simulink model "ExoskeletonControlModel"  (R2022b)
settings: Solver=ode3  StartTime=0.0  StopTime=inf  FixedStep=Ts  RelTol=1e-3
PreLoadFcn:
  | Ts_IO204 = 0.001;
  | 
  | if ~exist('Ts', 'var')
  | Ts = 0.001;
  | end
  | if ~exist('FPGA_Frequency', 'var')
  | FPGA_Frequency = 75000000;
  | end
  | 
  | ts_IO612 = 1e-3;
  | 
  | load('TargetReached.mat')
  | load('ActualPos_inc.mat')
model workspace (MAT data in the model file):
  DeltaData = timeseries
  DeltaData.DataInfo = tsdata.datametadata
  DeltaData.DataInfo.Interpolation = tsdata.interpolation
  DeltaData.DataInfo.Interpolation.Fhandle : function handle (value not decoded)
  DeltaData.DataInfo.Interpolation.Name = 'linear'
  DeltaData.TimeInfo = tsdata.timemetadata
  DeltaData.TimeInfo.Length = 30001
  DeltaData.TimeInfo.DuplicateTimes = 0
  DeltaData.TimeInfo.Increment_ = 0.001
  DeltaData.TimeInfo.Start_ = 0
  DeltaData.TimeInfo.Initialized = 1
  DeltaData.QualityInfo = tsdata.qualmetadata
  DeltaData.Data_ = [0 0 0 0 0 0 0 0 0 0 0 0 ... (180006 elements, 6x1x30001)]
  DeltaData.IsTimeFirst_ = 0
  EC45_deg2incs = 2276
  EC60_deg2inc = 5461
  EC90_deg2incs = 7111
  Enc2rad_18bit = 2.3968e-05
  Enc2rad_19bit = 1.1984e-05
  Enc2rad_20bit = 5.9921e-06
  GiulioModel = robotics.RigidBodyTree
  GiulioModel.TreeInternal = robotics.manip.internal.RigidBodyTree
  GiulioModel.TreeInternal.NumBodies = 7
  GiulioModel.TreeInternal.Base = robotics.manip.internal.RigidBody
  GiulioModel.TreeInternal.Base.Index = 0
  GiulioModel.TreeInternal.Base.NameInternal = 'base'
  GiulioModel.TreeInternal.Base.JointInternal = robotics.Joint
  GiulioModel.TreeInternal.Base.JointInternal.Type = 'fixed'
  GiulioModel.TreeInternal.Base.JointInternal.VelocityNumber = 0
  GiulioModel.TreeInternal.Base.JointInternal.PositionNumber = 0
  GiulioModel.TreeInternal.Base.JointInternal.MotionSubspace = [0; 0; 0; 0; 0; 0]
  GiulioModel.TreeInternal.Base.JointInternal.NameInternal = 'base_jnt'
  GiulioModel.TreeInternal.Base.ParentIndex = -1
  GiulioModel.TreeInternal.Base.ChildrenIndices = 1
  GiulioModel.TreeInternal.Base.MassInternal = 1
  GiulioModel.TreeInternal.Base.CenterOfMassInternal = [0 0 0]
  GiulioModel.TreeInternal.Base.InertiaInternal = [1  0  0; 0  1  0; 0  0  1]
  GiulioModel.TreeInternal.Base.SpatialInertia = [1  0  0  0  0  0; 0  1  0  0  0  0; 0  0  1  0  0  0; 0  0  0  1  0  0; 0  0  0  0  1  0; 0  0  0  0  0  1]
  GiulioModel.TreeInternal.Base.CollisionsInternal = robotics.manip.internal.CollisionSet
  GiulioModel.TreeInternal.Base.CollisionsInternal.MaxElements = 0
  GiulioModel.TreeInternal.FastVisualizationHelper = robotics.manip.internal.FastVisualizationHelper
  GiulioModel.TreeInternal.FastVisualizationHelper.IsUpdated = 0
  GiulioModel.TreeInternal.FastVisualizationHelper.MeshAndFrameOptions = [0 1 1]
  GiulioModel.TreeInternal.Gravity = [0 0 -9.81]
  GiulioModel.TreeInternal.Bodies{1} = robotics.manip.internal.RigidBody
  GiulioModel.TreeInternal.Bodies{1}.Index = 1
  GiulioModel.TreeInternal.Bodies{1}.NameInternal = 'body1'
  GiulioModel.TreeInternal.Bodies{1}.JointInternal = robotics.Joint
  GiulioModel.TreeInternal.Bodies{1}.JointInternal.Type = 'revolute'
  GiulioModel.TreeInternal.Bodies{1}.JointInternal.VelocityNumber = 1
  GiulioModel.TreeInternal.Bodies{1}.JointInternal.PositionNumber = 1
  GiulioModel.TreeInternal.Bodies{1}.JointInternal.MotionSubspace = [0; 0; 1; 0; 0; 0]
  GiulioModel.TreeInternal.Bodies{1}.JointInternal.InTree = 1
  GiulioModel.TreeInternal.Bodies{1}.JointInternal.JointToParentTransform = [1  0  0  0; 0  -1  -1.22464679915e-16  0; 0  1.22464679915e-16  -1  0; 0  0  0  1]
  GiulioModel.TreeInternal.Bodies{1}.JointInternal.NameInternal = 'jnt1'
  GiulioModel.TreeInternal.Bodies{1}.JointInternal.PositionLimitsInternal = [-0.733038285838 0.767246739177]
  GiulioModel.TreeInternal.Bodies{1}.JointInternal.JointAxisInternal = [0 0 1]
  GiulioModel.TreeInternal.Bodies{1}.ParentIndex = 0
  GiulioModel.TreeInternal.Bodies{1}.ChildrenIndices = [0 1]
  GiulioModel.TreeInternal.Bodies{1}.MassInternal = 2.789186
  GiulioModel.TreeInternal.Bodies{1}.CenterOfMassInternal = [5.3227185e-05 0.0036472886 -0.10689989]
  GiulioModel.TreeInternal.Bodies{1}.InertiaInternal = [0.010235641  5.0405441e-06  1.1186417e-05; 5.0405441e-06  0.011235393  0.0013102424; 1.1186417e-05  0.0013102424  0.0033699993]
  GiulioModel.TreeInternal.Bodies{1}.SpatialInertia = [0.010235641  5.0405441e-06  1.1186417e-05  0  0.29816367659  0.0101729663011; 5.0405441e-06  0.011235393  0.0013102424  -0.29816367659  0  -0.000148460519221; 1.1186417e-05  0.0013102424  0.0033699993  -0.0101729663011  0.000148460519221  0; 0  -0.29816367659  -0.0101729663011  2.789186  0  0; 0.29816367659  0  0.000148460519221  0  2.789186  0; 0.0101729663011  -0.000148460519221  0  0  0  2.789186]
  GiulioModel.TreeInternal.Bodies{1}.CollisionsInternal = robotics.manip.internal.CollisionSet
  GiulioModel.TreeInternal.Bodies{1}.CollisionsInternal.MaxElements = 0
  GiulioModel.TreeInternal.Bodies{2} = robotics.manip.internal.RigidBody
  GiulioModel.TreeInternal.Bodies{2}.Index = 2
  GiulioModel.TreeInternal.Bodies{2}.NameInternal = 'body2'
  GiulioModel.TreeInternal.Bodies{2}.JointInternal = robotics.Joint
  GiulioModel.TreeInternal.Bodies{2}.JointInternal.Type = 'revolute'
  GiulioModel.TreeInternal.Bodies{2}.JointInternal.VelocityNumber = 1
  GiulioModel.TreeInternal.Bodies{2}.JointInternal.PositionNumber = 1
  GiulioModel.TreeInternal.Bodies{2}.JointInternal.MotionSubspace = [0; 0; 1; 0; 0; 0]
  GiulioModel.TreeInternal.Bodies{2}.JointInternal.InTree = 1
  GiulioModel.TreeInternal.Bodies{2}.JointInternal.JointToParentTransform = [6.12323399574e-17  -1  0  0; 6.12323399574e-17  3.74939945665e-33  1  0.0092; -1  -6.12323399574e-17  6.12323399574e-17  -0.173338; 0  0  0  1]
  GiulioModel.TreeInternal.Bodies{2}.JointInternal.NameInternal = 'jnt2'
  GiulioModel.TreeInternal.Bodies{2}.JointInternal.PositionLimitsInternal = [-0.750491578358 0.304909020323]
  GiulioModel.TreeInternal.Bodies{2}.JointInternal.JointAxisInternal = [0 0 1]
  GiulioModel.TreeInternal.Bodies{2}.ParentIndex = 1
  GiulioModel.TreeInternal.Bodies{2}.ChildrenIndices = [0 0 1]
  GiulioModel.TreeInternal.Bodies{2}.MassInternal = 2.9144147
  GiulioModel.TreeInternal.Bodies{2}.CenterOfMassInternal = [0.0055350592 0.092636491 -0.046221487]
  GiulioModel.TreeInternal.Bodies{2}.InertiaInternal = [0.043969642  0.00022204015  0.00017139145; 0.00022204015  0.0030318204  0.0023833806; 0.00017139145  0.0023833806  0.043936348]
  GiulioModel.TreeInternal.Bodies{2}.SpatialInertia = [0.043969642  0.00022204015  0.00017139145  0  0.134708581169  0.269981151127; 0.00022204015  0.0030318204  0.0023833806  -0.134708581169  0  -0.0161314578979; 0.00017139145  0.0023833806  0.043936348  -0.269981151127  0.0161314578979  0; 0  -0.134708581169  -0.269981151127  2.9144147  0  0; 0.134708581169  0  0.0161314578979  0  2.9144147  0; 0.269981151127  -0.0161314578979  0  0  0  2.9144147]
  GiulioModel.TreeInternal.Bodies{2}.CollisionsInternal = robotics.manip.internal.CollisionSet
  GiulioModel.TreeInternal.Bodies{2}.CollisionsInternal.MaxElements = 0
  GiulioModel.TreeInternal.Bodies{3} = robotics.manip.internal.RigidBody
  GiulioModel.TreeInternal.Bodies{3}.Index = 3
  GiulioModel.TreeInternal.Bodies{3}.NameInternal = 'body3'
  GiulioModel.TreeInternal.Bodies{3}.JointInternal = robotics.Joint
  GiulioModel.TreeInternal.Bodies{3}.JointInternal.Type = 'revolute'
  GiulioModel.TreeInternal.Bodies{3}.JointInternal.VelocityNumber = 1
  GiulioModel.TreeInternal.Bodies{3}.JointInternal.PositionNumber = 1
  GiulioModel.TreeInternal.Bodies{3}.JointInternal.MotionSubspace = [0; 0; 1; 0; 0; 0]
  GiulioModel.TreeInternal.Bodies{3}.JointInternal.InTree = 1
  GiulioModel.TreeInternal.Bodies{3}.JointInternal.JointToParentTransform = [0.5  -0.866025403784  0  4.8059e-05; -0.813797681349  -0.469846310393  0.342020143326  0.19877; -0.296198132726  -0.171010071663  -0.939692620786  0.236333; 0  0  0  1]
  GiulioModel.TreeInternal.Bodies{3}.JointInternal.NameInternal = 'jnt3'
  GiulioModel.TreeInternal.Bodies{3}.JointInternal.PositionLimitsInternal = [-1.01874868439 1.26484010892]
  GiulioModel.TreeInternal.Bodies{3}.JointInternal.JointAxisInternal = [0 0 1]
  GiulioModel.TreeInternal.Bodies{3}.ParentIndex = 2
  GiulioModel.TreeInternal.Bodies{3}.ChildrenIndices = [0 0 0 1]
  GiulioModel.TreeInternal.Bodies{3}.MassInternal = 1.6194238
  GiulioModel.TreeInternal.Bodies{3}.CenterOfMassInternal = [0.00016105273 -0.083212269 0.18661296]
  GiulioModel.TreeInternal.Bodies{3}.InertiaInternal = [0.01950614  7.5954731e-05  0.00013309183; 7.5954731e-05  0.010143277  -0.0090554672; 0.00013309183  -0.0090554672  0.010093016]
  GiulioModel.TreeInternal.Bodies{3}.SpatialInertia = [0.01950614  7.5954731e-05  0.00013309183  0  -0.302205468812  -0.134755928871; 7.5954731e-05  0.010143277  -0.0090554672  0.302205468812  0  -0.000260812624017; 0.00013309183  -0.0090554672  0.010093016  0.134755928871  0.000260812624017  0; 0  0.302205468812  0.134755928871  1.6194238  0  0; -0.302205468812  0  0.000260812624017  0  1.6194238  0; -0.134755928871  -0.000260812624017  0  0  0  1.6194238]
  GiulioModel.TreeInternal.Bodies{3}.CollisionsInternal = robotics.manip.internal.CollisionSet
  GiulioModel.TreeInternal.Bodies{3}.CollisionsInternal.MaxElements = 0
  GiulioModel.TreeInternal.Bodies{4} = robotics.manip.internal.RigidBody
  GiulioModel.TreeInternal.Bodies{4}.Index = 4
  GiulioModel.TreeInternal.Bodies{4}.NameInternal = 'body4'
  GiulioModel.TreeInternal.Bodies{4}.JointInternal = robotics.Joint
  GiulioModel.TreeInternal.Bodies{4}.JointInternal.Type = 'revolute'
  GiulioModel.TreeInternal.Bodies{4}.JointInternal.VelocityNumber = 1
  GiulioModel.TreeInternal.Bodies{4}.JointInternal.PositionNumber = 1
  GiulioModel.TreeInternal.Bodies{4}.JointInternal.MotionSubspace = [0; 0; 1; 0; 0; 0]
  GiulioModel.TreeInternal.Bodies{4}.JointInternal.InTree = 1
  GiulioModel.TreeInternal.Bodies{4}.JointInternal.JointToParentTransform = [6.12323399574e-17  1  0  0; -0.51503807491  3.15369864939e-17  -0.857167300702  0; -0.857167300702  5.24863595569e-17  0.51503807491  0; 0  0  0  1]
  GiulioModel.TreeInternal.Bodies{4}.JointInternal.NameInternal = 'jnt4'
  GiulioModel.TreeInternal.Bodies{4}.JointInternal.PositionLimitsInternal = [-1.17120319455 1.61495315687]
  GiulioModel.TreeInternal.Bodies{4}.JointInternal.JointAxisInternal = [0 0 1]
  GiulioModel.TreeInternal.Bodies{4}.ParentIndex = 3
  GiulioModel.TreeInternal.Bodies{4}.ChildrenIndices = [0 0 0 0 1]
  GiulioModel.TreeInternal.Bodies{4}.MassInternal = 1.4377519
  GiulioModel.TreeInternal.Bodies{4}.CenterOfMassInternal = [0.00018140287 -0.064501229 0.11086441]
  GiulioModel.TreeInternal.Bodies{4}.InertiaInternal = [0.0085577992  7.3482248e-05  0.00013259917; 7.3482248e-05  0.0026666268  -0.0033203801; 0.00013259917  -0.0033203801  0.0064631147]
  GiulioModel.TreeInternal.Bodies{4}.SpatialInertia = [0.0085577992  7.3482248e-05  0.00013259917  0  -0.15939551612  -0.0927367645471; 7.3482248e-05  0.0026666268  -0.0033203801  0.15939551612  0  -0.000260812321008; 0.00013259917  -0.0033203801  0.0064631147  0.0927367645471  0.000260812321008  0; 0  0.15939551612  0.0927367645471  1.4377519  0  0; -0.15939551612  0  0.000260812321008  0  1.4377519  0; -0.0927367645471  -0.000260812321008  0  0  0  1.4377519]
  GiulioModel.TreeInternal.Bodies{4}.CollisionsInternal = robotics.manip.internal.CollisionSet
  GiulioModel.TreeInternal.Bodies{4}.CollisionsInternal.MaxElements = 0
  GiulioModel.TreeInternal.Bodies{5} = robotics.manip.internal.RigidBody
  GiulioModel.TreeInternal.Bodies{5}.Index = 5
  GiulioModel.TreeInternal.Bodies{5}.NameInternal = 'body5'
  GiulioModel.TreeInternal.Bodies{5}.JointInternal = robotics.Joint
  GiulioModel.TreeInternal.Bodies{5}.JointInternal.Type = 'revolute'
  GiulioModel.TreeInternal.Bodies{5}.JointInternal.VelocityNumber = 1
  GiulioModel.TreeInternal.Bodies{5}.JointInternal.PositionNumber = 1
  GiulioModel.TreeInternal.Bodies{5}.JointInternal.MotionSubspace = [0; 0; 1; 0; 0; 0]
  GiulioModel.TreeInternal.Bodies{5}.JointInternal.InTree = 1
  GiulioModel.TreeInternal.Bodies{5}.JointInternal.JointToParentTransform = [1  0  0  0; 0  0.5  -0.866025403784  0; 0  0.866025403784  0.5  0; 0  0  0  1]
  GiulioModel.TreeInternal.Bodies{5}.JointInternal.NameInternal = 'jnt5'
  GiulioModel.TreeInternal.Bodies{5}.JointInternal.PositionLimitsInternal = [-1.06098565229 1.93696640386]
  GiulioModel.TreeInternal.Bodies{5}.JointInternal.JointAxisInternal = [0 0 1]
  GiulioModel.TreeInternal.Bodies{5}.ParentIndex = 4
  GiulioModel.TreeInternal.Bodies{5}.ChildrenIndices = [0 0 0 0 0 1]
  GiulioModel.TreeInternal.Bodies{5}.MassInternal = 1.8609367
  GiulioModel.TreeInternal.Bodies{5}.CenterOfMassInternal = [0.00026237418 -0.14256313 0.098918728]
  GiulioModel.TreeInternal.Bodies{5}.InertiaInternal = [0.028991203  0.00016499917  1.6856413e-05; 0.00016499917  0.00160459  0.0013802979; 1.6856413e-05  0.0013802979  0.02826102]
  GiulioModel.TreeInternal.Bodies{5}.SpatialInertia = [0.028991203  0.00016499917  1.6856413e-05  0  -0.184081491253  -0.265300960684; 0.00016499917  0.00160459  0.0013802979  0.184081491253  0  -0.000488261740694; 1.6856413e-05  0.0013802979  0.02826102  0.265300960684  0.000488261740694  0; 0  0.184081491253  0.265300960684  1.8609367  0  0; -0.184081491253  0  0.000488261740694  0  1.8609367  0; -0.265300960684  -0.000488261740694  0  0  0  1.8609367]
  GiulioModel.TreeInternal.Bodies{5}.CollisionsInternal = robotics.manip.internal.CollisionSet
  GiulioModel.TreeInternal.Bodies{5}.CollisionsInternal.MaxElements = 0
  GiulioModel.TreeInternal.Bodies{6} = robotics.manip.internal.RigidBody
  GiulioModel.TreeInternal.Bodies{6}.Index = 6
  GiulioModel.TreeInternal.Bodies{6}.NameInternal = 'body6'
  GiulioModel.TreeInternal.Bodies{6}.JointInternal = robotics.Joint
  GiulioModel.TreeInternal.Bodies{6}.JointInternal.Type = 'revolute'
  GiulioModel.TreeInternal.Bodies{6}.JointInternal.VelocityNumber = 1
  GiulioModel.TreeInternal.Bodies{6}.JointInternal.PositionNumber = 1
  GiulioModel.TreeInternal.Bodies{6}.JointInternal.MotionSubspace = [0; 0; 1; 0; 0; 0]
  GiulioModel.TreeInternal.Bodies{6}.JointInternal.InTree = 1
  GiulioModel.TreeInternal.Bodies{6}.JointInternal.JointToParentTransform = [0  -1  6.4421e-06  -5.29259e-07; 1  0  -2.57e-08  -0.295612; 2.57e-08  6.4421e-06  1  -7.4581e-09; 0  0  0  1]
  GiulioModel.TreeInternal.Bodies{6}.JointInternal.NameInternal = 'jnt6'
  GiulioModel.TreeInternal.Bodies{6}.JointInternal.PositionLimitsInternal = [-1.53616899444 0.741415866247]
  GiulioModel.TreeInternal.Bodies{6}.JointInternal.JointAxisInternal = [0 0 1]
  GiulioModel.TreeInternal.Bodies{6}.ParentIndex = 5
  GiulioModel.TreeInternal.Bodies{6}.ChildrenIndices = [0 0 0 0 0 0 1]
  GiulioModel.TreeInternal.Bodies{6}.MassInternal = 1.3019553
  GiulioModel.TreeInternal.Bodies{6}.CenterOfMassInternal = [0.00026780979 -0.0546904 0.068766033]
  GiulioModel.TreeInternal.Bodies{6}.InertiaInternal = [0.0054780511  2.1188231e-06  2.1188231e-06; 2.1188231e-06  0.00084113267  -0.00058999652; 2.1188231e-06  -0.00058999652  0.0057331244]
  GiulioModel.TreeInternal.Bodies{6}.SpatialInertia = [0.0054780511  2.1188231e-06  2.1188231e-06  0  -0.0895303011243  -0.0712044561391; 2.1188231e-06  0.00084113267  -0.00058999652  0.0895303011243  0  -0.000348676375482; 2.1188231e-06  -0.00058999652  0.0057331244  0.0712044561391  0.000348676375482  0; 0  0.0895303011243  0.0712044561391  1.3019553  0  0; -0.0895303011243  0  0.000348676375482  0  1.3019553  0; -0.0712044561391  -0.000348676375482  0  0  0  1.3019553]
  GiulioModel.TreeInternal.Bodies{6}.CollisionsInternal = robotics.manip.internal.CollisionSet
  GiulioModel.TreeInternal.Bodies{6}.CollisionsInternal.MaxElements = 0
  GiulioModel.TreeInternal.Bodies{7} = robotics.manip.internal.RigidBody
  GiulioModel.TreeInternal.Bodies{7}.Index = 7
  GiulioModel.TreeInternal.Bodies{7}.NameInternal = 'endeffector'
  GiulioModel.TreeInternal.Bodies{7}.JointInternal = robotics.Joint
  GiulioModel.TreeInternal.Bodies{7}.JointInternal.Type = 'fixed'
  GiulioModel.TreeInternal.Bodies{7}.JointInternal.VelocityNumber = 0
  GiulioModel.TreeInternal.Bodies{7}.JointInternal.PositionNumber = 0
  GiulioModel.TreeInternal.Bodies{7}.JointInternal.MotionSubspace = [0; 0; 0; 0; 0; 0]
  GiulioModel.TreeInternal.Bodies{7}.JointInternal.InTree = 1
  GiulioModel.TreeInternal.Bodies{7}.JointInternal.JointToParentTransform = [1  0  0  0; 0  1  0  -0.15; 0  0  1  0.080356; 0  0  0  1]
  GiulioModel.TreeInternal.Bodies{7}.JointInternal.NameInternal = 'endeffector_jnt'
  GiulioModel.TreeInternal.Bodies{7}.ParentIndex = 6
  GiulioModel.TreeInternal.Bodies{7}.ChildrenIndices = [0 0 0 0 0 0]
  GiulioModel.TreeInternal.Bodies{7}.MassInternal = 0
  GiulioModel.TreeInternal.Bodies{7}.CenterOfMassInternal = [0 0 0]
  GiulioModel.TreeInternal.Bodies{7}.InertiaInternal = [1  0  0; 0  1  0; 0  0  1]
  GiulioModel.TreeInternal.Bodies{7}.SpatialInertia = [1  0  0  0  0  0; 0  1  0  0  0  0; 0  0  1  0  0  0; 0  0  0  0  0  0; 0  0  0  0  0  0; 0  0  0  0  0  0]
  GiulioModel.TreeInternal.Bodies{7}.CollisionsInternal = robotics.manip.internal.CollisionSet
  GiulioModel.TreeInternal.Bodies{7}.CollisionsInternal.MaxElements = 0
  GiulioModel.TreeInternal.NumNonFixedBodies = 6
  GiulioModel.TreeInternal.PositionNumber = 6
  GiulioModel.TreeInternal.VelocityNumber = 6
  GiulioModel.TreeInternal.PositionDoFMap = [1  1; 2  2; 3  3; 4  4; 5  5; 6  6; 0  -1]
  GiulioModel.TreeInternal.VelocityDoFMap = [1  1; 2  2; 3  3; 4  4; 5  5; 6  6; 0  -1]
  GiulioModel.TreeInternal.MaxNumBodies = 7
  GiulioModel.TreeInternal.MaxNameLength = 200
  GiulioModel.TreeInternal.MaxJointPositionNumber = 7
  GiulioModel.TreeInternal.VisualizationInfo = robotics.manip.internal.VisualizationInfo
  GiulioModel.TreeInternal.VisualizationInfo.ShowTag = 'DO_NOT_EDIT_OUhUD'
  GiulioModel.TreeInternal.DataFormatInternal = 'struct'
  Giulio_Spheric_model = robotics.RigidBodyTree
  Giulio_Spheric_model.TreeInternal = robotics.manip.internal.RigidBodyTree
  Giulio_Spheric_model.TreeInternal.NumBodies = 7
  Giulio_Spheric_model.TreeInternal.Base = robotics.manip.internal.RigidBody
  Giulio_Spheric_model.TreeInternal.Base.Index = 0
  Giulio_Spheric_model.TreeInternal.Base.NameInternal = 'base'
  Giulio_Spheric_model.TreeInternal.Base.JointInternal = robotics.Joint
  Giulio_Spheric_model.TreeInternal.Base.JointInternal.Type = 'fixed'
  Giulio_Spheric_model.TreeInternal.Base.JointInternal.VelocityNumber = 0
  Giulio_Spheric_model.TreeInternal.Base.JointInternal.PositionNumber = 0
  Giulio_Spheric_model.TreeInternal.Base.JointInternal.MotionSubspace = [0; 0; 0; 0; 0; 0]
  Giulio_Spheric_model.TreeInternal.Base.JointInternal.NameInternal = 'base_jnt'
  Giulio_Spheric_model.TreeInternal.Base.ParentIndex = -1
  Giulio_Spheric_model.TreeInternal.Base.ChildrenIndices = [1 0 0 1]
  Giulio_Spheric_model.TreeInternal.Base.MassInternal = 1
  Giulio_Spheric_model.TreeInternal.Base.CenterOfMassInternal = [0 0 0]
  Giulio_Spheric_model.TreeInternal.Base.InertiaInternal = [1  0  0; 0  1  0; 0  0  1]
  Giulio_Spheric_model.TreeInternal.Base.SpatialInertia = [1  0  0  0  0  0; 0  1  0  0  0  0; 0  0  1  0  0  0; 0  0  0  1  0  0; 0  0  0  0  1  0; 0  0  0  0  0  1]
  Giulio_Spheric_model.TreeInternal.Base.CollisionsInternal = robotics.manip.internal.CollisionSet
  Giulio_Spheric_model.TreeInternal.Base.CollisionsInternal.MaxElements = 0
  Giulio_Spheric_model.TreeInternal.FastVisualizationHelper = robotics.manip.internal.FastVisualizationHelper
  Giulio_Spheric_model.TreeInternal.FastVisualizationHelper.IsUpdated = 0
  Giulio_Spheric_model.TreeInternal.FastVisualizationHelper.MeshAndFrameOptions = [0 1 1]
  Giulio_Spheric_model.TreeInternal.Gravity = [0 0 -9.81]
  Giulio_Spheric_model.TreeInternal.Bodies{1} = robotics.manip.internal.RigidBody
  Giulio_Spheric_model.TreeInternal.Bodies{1}.Index = 1
  Giulio_Spheric_model.TreeInternal.Bodies{1}.NameInternal = 'body0'
  Giulio_Spheric_model.TreeInternal.Bodies{1}.JointInternal = robotics.Joint
  Giulio_Spheric_model.TreeInternal.Bodies{1}.JointInternal.Type = 'fixed'
  Giulio_Spheric_model.TreeInternal.Bodies{1}.JointInternal.VelocityNumber = 0
  Giulio_Spheric_model.TreeInternal.Bodies{1}.JointInternal.PositionNumber = 0
  Giulio_Spheric_model.TreeInternal.Bodies{1}.JointInternal.MotionSubspace = [0; 0; 0; 0; 0; 0]
  Giulio_Spheric_model.TreeInternal.Bodies{1}.JointInternal.InTree = 1
  Giulio_Spheric_model.TreeInternal.Bodies{1}.JointInternal.JointToParentTransform = [0  -1  0  0; -1  0  0  0; 0  0  -1  0; 0  0  0  1]
  Giulio_Spheric_model.TreeInternal.Bodies{1}.JointInternal.NameInternal = 'jnt0'
  Giulio_Spheric_model.TreeInternal.Bodies{1}.ParentIndex = 0
  Giulio_Spheric_model.TreeInternal.Bodies{1}.ChildrenIndices = [0 1]
  Giulio_Spheric_model.TreeInternal.Bodies{1}.MassInternal = 1
  Giulio_Spheric_model.TreeInternal.Bodies{1}.CenterOfMassInternal = [0 0 0]
  Giulio_Spheric_model.TreeInternal.Bodies{1}.InertiaInternal = [1  0  0; 0  1  0; 0  0  1]
  Giulio_Spheric_model.TreeInternal.Bodies{1}.SpatialInertia = [1  0  0  0  0  0; 0  1  0  0  0  0; 0  0  1  0  0  0; 0  0  0  1  0  0; 0  0  0  0  1  0; 0  0  0  0  0  1]
  Giulio_Spheric_model.TreeInternal.Bodies{1}.CollisionsInternal = robotics.manip.internal.CollisionSet
  Giulio_Spheric_model.TreeInternal.Bodies{1}.CollisionsInternal.MaxElements = 0
  Giulio_Spheric_model.TreeInternal.Bodies{2} = robotics.manip.internal.RigidBody
  Giulio_Spheric_model.TreeInternal.Bodies{2}.Index = 2
  Giulio_Spheric_model.TreeInternal.Bodies{2}.NameInternal = 'body_yaw'
  Giulio_Spheric_model.TreeInternal.Bodies{2}.JointInternal = robotics.Joint
  Giulio_Spheric_model.TreeInternal.Bodies{2}.JointInternal.Type = 'fixed'
  Giulio_Spheric_model.TreeInternal.Bodies{2}.JointInternal.VelocityNumber = 0
  Giulio_Spheric_model.TreeInternal.Bodies{2}.JointInternal.PositionNumber = 0
  Giulio_Spheric_model.TreeInternal.Bodies{2}.JointInternal.MotionSubspace = [0; 0; 0; 0; 0; 0]
  Giulio_Spheric_model.TreeInternal.Bodies{2}.JointInternal.InTree = 1
  Giulio_Spheric_model.TreeInternal.Bodies{2}.JointInternal.JointToParentTransform = [0.9778  0.2096  0  0; -0.2096  0.9778  0  0; 0  0  1  0; 0  0  0  1]
  Giulio_Spheric_model.TreeInternal.Bodies{2}.JointInternal.NameInternal = 'jnty'
  Giulio_Spheric_model.TreeInternal.Bodies{2}.ParentIndex = 1
  Giulio_Spheric_model.TreeInternal.Bodies{2}.ChildrenIndices = [0 0 1]
  Giulio_Spheric_model.TreeInternal.Bodies{2}.MassInternal = 1
  Giulio_Spheric_model.TreeInternal.Bodies{2}.CenterOfMassInternal = [0 0 0]
  Giulio_Spheric_model.TreeInternal.Bodies{2}.InertiaInternal = [1  0  0; 0  1  0; 0  0  1]
  Giulio_Spheric_model.TreeInternal.Bodies{2}.SpatialInertia = [1  0  0  0  0  0; 0  1  0  0  0  0; 0  0  1  0  0  0; 0  0  0  1  0  0; 0  0  0  0  1  0; 0  0  0  0  0  1]
  Giulio_Spheric_model.TreeInternal.Bodies{2}.CollisionsInternal = robotics.manip.internal.CollisionSet
  Giulio_Spheric_model.TreeInternal.Bodies{2}.CollisionsInternal.MaxElements = 0
  Giulio_Spheric_model.TreeInternal.Bodies{3} = robotics.manip.internal.RigidBody
  Giulio_Spheric_model.TreeInternal.Bodies{3}.Index = 3
  Giulio_Spheric_model.TreeInternal.Bodies{3}.NameInternal = 'body_pitch'
  Giulio_Spheric_model.TreeInternal.Bodies{3}.JointInternal = robotics.Joint
  Giulio_Spheric_model.TreeInternal.Bodies{3}.JointInternal.Type = 'fixed'
  Giulio_Spheric_model.TreeInternal.Bodies{3}.JointInternal.VelocityNumber = 0
  Giulio_Spheric_model.TreeInternal.Bodies{3}.JointInternal.PositionNumber = 0
  Giulio_Spheric_model.TreeInternal.Bodies{3}.JointInternal.MotionSubspace = [0; 0; 0; 0; 0; 0]
  Giulio_Spheric_model.TreeInternal.Bodies{3}.JointInternal.InTree = 1
  Giulio_Spheric_model.TreeInternal.Bodies{3}.JointInternal.JointToParentTransform = [0.454  0  -0.891  0; 0  1  0  0; 0.891  0  0.454  0; 0  0  0  1]
  Giulio_Spheric_model.TreeInternal.Bodies{3}.JointInternal.NameInternal = 'jntpitch'
  Giulio_Spheric_model.TreeInternal.Bodies{3}.ParentIndex = 2
  Giulio_Spheric_model.TreeInternal.Bodies{3}.ChildrenIndices = [0 0]
  Giulio_Spheric_model.TreeInternal.Bodies{3}.MassInternal = 1
  Giulio_Spheric_model.TreeInternal.Bodies{3}.CenterOfMassInternal = [0 0 0]
  Giulio_Spheric_model.TreeInternal.Bodies{3}.InertiaInternal = [1  0  0; 0  1  0; 0  0  1]
  Giulio_Spheric_model.TreeInternal.Bodies{3}.SpatialInertia = [1  0  0  0  0  0; 0  1  0  0  0  0; 0  0  1  0  0  0; 0  0  0  1  0  0; 0  0  0  0  1  0; 0  0  0  0  0  1]
  Giulio_Spheric_model.TreeInternal.Bodies{3}.CollisionsInternal = robotics.manip.internal.CollisionSet
  Giulio_Spheric_model.TreeInternal.Bodies{3}.CollisionsInternal.MaxElements = 0
  Giulio_Spheric_model.TreeInternal.Bodies{4} = robotics.manip.internal.RigidBody
  Giulio_Spheric_model.TreeInternal.Bodies{4}.Index = 4
  Giulio_Spheric_model.TreeInternal.Bodies{4}.NameInternal = 'body3'
  Giulio_Spheric_model.TreeInternal.Bodies{4}.JointInternal = robotics.Joint
  Giulio_Spheric_model.TreeInternal.Bodies{4}.JointInternal.Type = 'revolute'
  Giulio_Spheric_model.TreeInternal.Bodies{4}.JointInternal.VelocityNumber = 1
  Giulio_Spheric_model.TreeInternal.Bodies{4}.JointInternal.PositionNumber = 1
  Giulio_Spheric_model.TreeInternal.Bodies{4}.JointInternal.MotionSubspace = [0; 0; 1; 0; 0; 0]
  Giulio_Spheric_model.TreeInternal.Bodies{4}.JointInternal.InTree = 1
  Giulio_Spheric_model.TreeInternal.Bodies{4}.JointInternal.JointToParentTransform = [0.8138  0.4698  -0.342  0; 0.2962  0.171  0.9397  0; 0.5  -0.866  0  0; 0  0  0  1]
  Giulio_Spheric_model.TreeInternal.Bodies{4}.JointInternal.NameInternal = 'jnt3'
  Giulio_Spheric_model.TreeInternal.Bodies{4}.JointInternal.PositionLimitsInternal = [-1.01874868439 1.26484010892]
  Giulio_Spheric_model.TreeInternal.Bodies{4}.JointInternal.JointAxisInternal = [0 0 1]
  Giulio_Spheric_model.TreeInternal.Bodies{4}.ParentIndex = 0
  Giulio_Spheric_model.TreeInternal.Bodies{4}.ChildrenIndices = [0 0 0 0 1]
  Giulio_Spheric_model.TreeInternal.Bodies{4}.MassInternal = 1.6194238
  Giulio_Spheric_model.TreeInternal.Bodies{4}.CenterOfMassInternal = [0.00016105273 -0.083212269 0.18661296]
  Giulio_Spheric_model.TreeInternal.Bodies{4}.InertiaInternal = [0.01950614  7.5954731e-05  0.00013309183; 7.5954731e-05  0.010143277  -0.0090554672; 0.00013309183  -0.0090554672  0.010093016]
  Giulio_Spheric_model.TreeInternal.Bodies{4}.SpatialInertia = [0.01950614  7.5954731e-05  0.00013309183  0  -0.302205468812  -0.134755928871; 7.5954731e-05  0.010143277  -0.0090554672  0.302205468812  0  -0.000260812624017; 0.00013309183  -0.0090554672  0.010093016  0.134755928871  0.000260812624017  0; 0  0.302205468812  0.134755928871  1.6194238  0  0; -0.302205468812  0  0.000260812624017  0  1.6194238  0; -0.134755928871  -0.000260812624017  0  0  0  1.6194238]
  Giulio_Spheric_model.TreeInternal.Bodies{4}.CollisionsInternal = robotics.manip.internal.CollisionSet
  Giulio_Spheric_model.TreeInternal.Bodies{4}.CollisionsInternal.MaxElements = 0
  Giulio_Spheric_model.TreeInternal.Bodies{5} = robotics.manip.internal.RigidBody
  Giulio_Spheric_model.TreeInternal.Bodies{5}.Index = 5
  Giulio_Spheric_model.TreeInternal.Bodies{5}.NameInternal = 'body4'
  Giulio_Spheric_model.TreeInternal.Bodies{5}.JointInternal = robotics.Joint
  Giulio_Spheric_model.TreeInternal.Bodies{5}.JointInternal.Type = 'revolute'
  Giulio_Spheric_model.TreeInternal.Bodies{5}.JointInternal.VelocityNumber = 1
  Giulio_Spheric_model.TreeInternal.Bodies{5}.JointInternal.PositionNumber = 1
  Giulio_Spheric_model.TreeInternal.Bodies{5}.JointInternal.MotionSubspace = [0; 0; 1; 0; 0; 0]
  Giulio_Spheric_model.TreeInternal.Bodies{5}.JointInternal.InTree = 1
  Giulio_Spheric_model.TreeInternal.Bodies{5}.JointInternal.JointToParentTransform = [6.12323399574e-17  1  0  0; -0.51503807491  3.15369864939e-17  -0.857167300702  0; -0.857167300702  5.24863595569e-17  0.51503807491  0; 0  0  0  1]
  Giulio_Spheric_model.TreeInternal.Bodies{5}.JointInternal.NameInternal = 'jnt4'
  Giulio_Spheric_model.TreeInternal.Bodies{5}.JointInternal.PositionLimitsInternal = [-1.17120319455 1.61495315687]
  Giulio_Spheric_model.TreeInternal.Bodies{5}.JointInternal.JointAxisInternal = [0 0 1]
  Giulio_Spheric_model.TreeInternal.Bodies{5}.ParentIndex = 4
  Giulio_Spheric_model.TreeInternal.Bodies{5}.ChildrenIndices = [0 0 0 0 0 1]
  Giulio_Spheric_model.TreeInternal.Bodies{5}.MassInternal = 1.4377519
  Giulio_Spheric_model.TreeInternal.Bodies{5}.CenterOfMassInternal = [0.00018140287 -0.064501229 0.11086441]
  Giulio_Spheric_model.TreeInternal.Bodies{5}.InertiaInternal = [0.0085577992  7.3482248e-05  0.00013259917; 7.3482248e-05  0.0026666268  -0.0033203801; 0.00013259917  -0.0033203801  0.0064631147]
  Giulio_Spheric_model.TreeInternal.Bodies{5}.SpatialInertia = [0.0085577992  7.3482248e-05  0.00013259917  0  -0.15939551612  -0.0927367645471; 7.3482248e-05  0.0026666268  -0.0033203801  0.15939551612  0  -0.000260812321008; 0.00013259917  -0.0033203801  0.0064631147  0.0927367645471  0.000260812321008  0; 0  0.15939551612  0.0927367645471  1.4377519  0  0; -0.15939551612  0  0.000260812321008  0  1.4377519  0; -0.0927367645471  -0.000260812321008  0  0  0  1.4377519]
  Giulio_Spheric_model.TreeInternal.Bodies{5}.CollisionsInternal = robotics.manip.internal.CollisionSet
  Giulio_Spheric_model.TreeInternal.Bodies{5}.CollisionsInternal.MaxElements = 0
  Giulio_Spheric_model.TreeInternal.Bodies{6} = robotics.manip.internal.RigidBody
  Giulio_Spheric_model.TreeInternal.Bodies{6}.Index = 6
  Giulio_Spheric_model.TreeInternal.Bodies{6}.NameInternal = 'body5'
  Giulio_Spheric_model.TreeInternal.Bodies{6}.JointInternal = robotics.Joint
  Giulio_Spheric_model.TreeInternal.Bodies{6}.JointInternal.Type = 'revolute'
  Giulio_Spheric_model.TreeInternal.Bodies{6}.JointInternal.VelocityNumber = 1
  Giulio_Spheric_model.TreeInternal.Bodies{6}.JointInternal.PositionNumber = 1
  Giulio_Spheric_model.TreeInternal.Bodies{6}.JointInternal.MotionSubspace = [0; 0; 1; 0; 0; 0]
  Giulio_Spheric_model.TreeInternal.Bodies{6}.JointInternal.InTree = 1
  Giulio_Spheric_model.TreeInternal.Bodies{6}.JointInternal.JointToParentTransform = [1  0  0  0; 0  0.5  -0.866025403784  0; 0  0.866025403784  0.5  0; 0  0  0  1]
  Giulio_Spheric_model.TreeInternal.Bodies{6}.JointInternal.NameInternal = 'jnt5'
  Giulio_Spheric_model.TreeInternal.Bodies{6}.JointInternal.PositionLimitsInternal = [-1.06098565229 1.93696640386]
  Giulio_Spheric_model.TreeInternal.Bodies{6}.JointInternal.JointAxisInternal = [0 0 1]
  Giulio_Spheric_model.TreeInternal.Bodies{6}.ParentIndex = 5
  Giulio_Spheric_model.TreeInternal.Bodies{6}.ChildrenIndices = [0 0 0 0 0 0 1]
  Giulio_Spheric_model.TreeInternal.Bodies{6}.MassInternal = 1.8609367
  Giulio_Spheric_model.TreeInternal.Bodies{6}.CenterOfMassInternal = [0.00026237418 -0.14256313 0.098918728]
  Giulio_Spheric_model.TreeInternal.Bodies{6}.InertiaInternal = [0.028991203  0.00016499917  1.6856413e-05; 0.00016499917  0.00160459  0.0013802979; 1.6856413e-05  0.0013802979  0.02826102]
  Giulio_Spheric_model.TreeInternal.Bodies{6}.SpatialInertia = [0.028991203  0.00016499917  1.6856413e-05  0  -0.184081491253  -0.265300960684; 0.00016499917  0.00160459  0.0013802979  0.184081491253  0  -0.000488261740694; 1.6856413e-05  0.0013802979  0.02826102  0.265300960684  0.000488261740694  0; 0  0.184081491253  0.265300960684  1.8609367  0  0; -0.184081491253  0  0.000488261740694  0  1.8609367  0; -0.265300960684  -0.000488261740694  0  0  0  1.8609367]
  Giulio_Spheric_model.TreeInternal.Bodies{6}.CollisionsInternal = robotics.manip.internal.CollisionSet
  Giulio_Spheric_model.TreeInternal.Bodies{6}.CollisionsInternal.MaxElements = 0
  Giulio_Spheric_model.TreeInternal.Bodies{7} = robotics.manip.internal.RigidBody
  Giulio_Spheric_model.TreeInternal.Bodies{7}.Index = 7
  Giulio_Spheric_model.TreeInternal.Bodies{7}.NameInternal = 'endeffector'
  Giulio_Spheric_model.TreeInternal.Bodies{7}.JointInternal = robotics.Joint
  Giulio_Spheric_model.TreeInternal.Bodies{7}.JointInternal.Type = 'fixed'
  Giulio_Spheric_model.TreeInternal.Bodies{7}.JointInternal.VelocityNumber = 0
  Giulio_Spheric_model.TreeInternal.Bodies{7}.JointInternal.PositionNumber = 0
  Giulio_Spheric_model.TreeInternal.Bodies{7}.JointInternal.MotionSubspace = [0; 0; 0; 0; 0; 0]
  Giulio_Spheric_model.TreeInternal.Bodies{7}.JointInternal.InTree = 1
  Giulio_Spheric_model.TreeInternal.Bodies{7}.JointInternal.JointToParentTransform = [0  0  -1  0; -1  0  0  -0.295612; 0  1  0  0; 0  0  0  1]
  Giulio_Spheric_model.TreeInternal.Bodies{7}.JointInternal.NameInternal = 'endeffector_jnt'
  Giulio_Spheric_model.TreeInternal.Bodies{7}.ParentIndex = 6
  Giulio_Spheric_model.TreeInternal.Bodies{7}.ChildrenIndices = [0 0 0 0 0 0]
  Giulio_Spheric_model.TreeInternal.Bodies{7}.MassInternal = 0
  Giulio_Spheric_model.TreeInternal.Bodies{7}.CenterOfMassInternal = [0 0 0]
  Giulio_Spheric_model.TreeInternal.Bodies{7}.InertiaInternal = [1  0  0; 0  1  0; 0  0  1]
  Giulio_Spheric_model.TreeInternal.Bodies{7}.SpatialInertia = [1  0  0  0  0  0; 0  1  0  0  0  0; 0  0  1  0  0  0; 0  0  0  0  0  0; 0  0  0  0  0  0; 0  0  0  0  0  0]
  Giulio_Spheric_model.TreeInternal.Bodies{7}.CollisionsInternal = robotics.manip.internal.CollisionSet
  Giulio_Spheric_model.TreeInternal.Bodies{7}.CollisionsInternal.MaxElements = 0
  Giulio_Spheric_model.TreeInternal.NumNonFixedBodies = 3
  Giulio_Spheric_model.TreeInternal.PositionNumber = 3
  Giulio_Spheric_model.TreeInternal.VelocityNumber = 3
  Giulio_Spheric_model.TreeInternal.PositionDoFMap = [0  -1; 0  -1; 0  -1; 1  1; 2  2; 3  3; 0  -1]
  Giulio_Spheric_model.TreeInternal.VelocityDoFMap = [0  -1; 0  -1; 0  -1; 1  1; 2  2; 3  3; 0  -1]
  Giulio_Spheric_model.TreeInternal.MaxNumBodies = 7
  Giulio_Spheric_model.TreeInternal.MaxNameLength = 200
  Giulio_Spheric_model.TreeInternal.MaxJointPositionNumber = 7
  Giulio_Spheric_model.TreeInternal.VisualizationInfo = robotics.manip.internal.VisualizationInfo
  Giulio_Spheric_model.TreeInternal.VisualizationInfo.ShowTag = 'DO_NOT_EDIT_gr7XX'
  Giulio_Spheric_model.TreeInternal.DataFormatInternal = 'struct'
  Offset1_ticks = 571315
  Offset2_ticks = 590938.9928
  Offset3_ticks = 457912.8279
  Offset4_ticks = 482293.9763
  Offset5_ticks = 598735.9316
  Offset_M1 = 1.12645499896
  Offset_M2 = 4.02728553608
  Offset_M3 = 5.48587511336
  Offset_M4 = 2.03717511516
  Offset_M5 = 4.4996674016
  T1_Nm.time = [0.002125 0.003375 0.004125 0.0055 0.006125 0.007375 0.008125 0.009375 0.010125 0.011375 0.012125 0.013375 ... (119999 elements, 119999x1)]
  T1_Nm.signals.values = [-0.0898684700197 -0.0898684700197 -0.0946888340762 -0.104329562189 -0.104329562189 -0.113970290302 -0.118790654359 -0.128431382472 -0.123611018415 -0.134858534547 -0.138072110585 -0.14449926266 ... (119999 elements, 119999x1)]
  T1_Nm.signals.dimensione = 1
  T2_Nm.time = [0.002125 0.003375 0.004125 0.0055 0.006125 0.007375 0.008125 0.009375 0.010125 0.011375 0.012125 0.013375 ... (119999 elements, 119999x1)]
  T2_Nm.signals.values = [0.485488545273 0.488371356072 0.487218231753 0.490101042552 0.495290101991 0.49874947495 0.502785410069 0.508551031668 0.514316653267 0.516622901907 0.524694772145 0.526424458624 ... (119999 elements, 119999x1)]
  T2_Nm.signals.dimensione = 1
  TBmodel : robotics.RigidBodyTree (value not decoded)
  Ts = 0.002
  Xg.time = [0 0.12012012012 0.24024024024 0.36036036036 0.48048048048 0.600600600601 0.720720720721 0.840840840841 0.960960960961 1.08108108108 1.2012012012 1.32132132132 ... (1000 elements, 1x1000)]
  Xg.signals.values = [-0.0136648258725 -0.0136648258725 -0.0136648258725 -0.0136648258725 -0.0136648258725 -0.0136648258725 -0.0136648258725 -0.0136648258725 -0.0136648258725 -0.0136648258725 -0.0136648258725 -0.0136648258725 ... (1000 elements, 1000x1)]
  Xg.signals.dimensione = 1
  Yg.time = [0 0.12012012012 0.24024024024 0.36036036036 0.48048048048 0.600600600601 0.720720720721 0.840840840841 0.960960960961 1.08108108108 1.2012012012 1.32132132132 ... (1000 elements, 1x1000)]
  Yg.signals.values = [-0.138973252652 -0.138973252652 -0.138973252652 -0.138973252652 -0.138973252652 -0.138973252652 -0.138973252652 -0.138973252652 -0.138973252652 -0.138973252652 -0.138973252652 -0.138973252652 ... (1000 elements, 1000x1)]
  Yg.signals.dimensione = 1
  Zg.time = [0 0.12012012012 0.24024024024 0.36036036036 0.48048048048 0.600600600601 0.720720720721 0.840840840841 0.960960960961 1.08108108108 1.2012012012 1.32132132132 ... (1000 elements, 1x1000)]
  Zg.signals.values = [0.446887320928 0.446887320928 0.446887320928 0.446887320928 0.446887320928 0.446887320928 0.446887320928 0.446887320928 0.446887320928 0.446887320928 0.446887320928 0.446887320928 ... (1000 elements, 1000x1)]
  Zg.signals.dimensione = 1
  a2 = 0.27
  change_variable = 0
  d1 = [0 0 0 0 0 0 0 0 0 0 0 0 ... (30001 elements, 30001x1)]
  d1_1 = 0.21074
  d2 = [0 0 0 0 0 0 0 0 0 0 0 0 ... (30001 elements, 30001x1)]
  d2_1 = 0.04864
  d3 = [0 0 0 0 0 0 0 0 0 0 0 0 ... (30001 elements, 30001x1)]
  d4 = [0 0 0 0 0 0 0 0 0 0 0 0 ... (30001 elements, 30001x1)]
  d5 = [0 0 0 0 0 0 0 0 0 0 0 0 ... (30001 elements, 30001x1)]
  d6 = [0 0 0 0 0 0 0 0 0 0 0 0 ... (30001 elements, 30001x1)]
  ee_x = -0.2852
  ee_y = -0.3683
  ee_z = -0.0386
  enc2rad_EC45 = 7.6699e-06
  enc2rad_EC90 = 2.3969e-05
  k1_Nm_ticks = 0.00923
  k2_Nm_ticks = 0.0257
  k3_Nm_ticks = 0.00692
  k4_Nm_ticks = 0.00729
  k5_Nm_ticks = 0.00641
  lower_lim_m1 = -330000
  lower_lim_m2 = -235302
  lower_lim_m3 = -132865
  lower_lim_m4 = -152732
  lower_lim_m5 = -138363
  lower_lim_m6 = -200325
  m1 = 2.441408578
  m2 = 3.750007
  m3 = 1.56250298
  m4 = 1.56250298
  m5 = 1.56250298
  m6 = 1.56250298
  n_oversampling = 8
  offset_sea_1 = 0.5547
  offset_sea_2 = 2.8595
  offset_sea_3 = 3.5058
  offset_sea_4 = 2.8586
  offset_sea_5 = 2.8736
  params.AKSIM.commandString = [51; 51]
  params.AKSIM.nBytesSent = [1 1]
  params.AKSIM.myg = 2
  pos_th_neg = -180000
  pos_th_pos = 180000
  q1 = -1819347
  q2 = -196752
  q3 = -596465
  q4 = -556807
  q5 = -573932
  q6 = -489063
  sine = [0 0.187999937334 0.751998997352 1.69199492401 3.0079839574 4.6999608335 6.76791878442 9.21184953835 12.0317433196 15.2275888485 18.7993733417 22.7470825122 ... (12501 elements, 12501x1)]
  start.time = [0 0.12012012012 0.24024024024 0.36036036036 0.48048048048 0.600600600601 0.720720720721 0.840840840841 0.960960960961 1.08108108108 1.2012012012 1.32132132132 ... (1000 elements, 1x1000)]
  start.signals.values = [1 0 0 0 0 0 0 0 0 0 0 0 ... (1000 elements, 1000x1)]
  start.signals.dimensione = 1
  switch_admittance = 1
  t1.time = [0 0.001 0.002 0.003 0.004 0.005 0.006 0.007 0.008 0.009 0.01 0.011 ... (10001 elements, 1x10001)]
  t1.signals.values = [-12 -12 -12 -12 -12 -12 -12 -12 -12 -12 -12 -12 ... (10001 elements, 10001x1)]
  t1.signals.dimensione = 1
  t2.time = [0 0.001 0.002 0.003 0.004 0.005 0.006 0.007 0.008 0.009 0.01 0.011 ... (10001 elements, 1x10001)]
  t2.signals.values = [-9 -9 -9 -9 -9 -9 -9 -9 -9 -9 -9 -9 ... (10001 elements, 10001x1)]
  t2.signals.dimensione = 1
  torsionalStiffnes_M1 = 384.88
  torsionalStiffnes_M2 = 1500
  torsionalStiffnes_M3 = 901.97
  torsionalStiffnes_M4 = 950.86
  torsionalStiffnes_M5 = 930
  torsionalStiffnes_M6 = 914
  upper_lim_m1 = 340000
  upper_lim_m2 = 95467
  upper_lim_m3 = 164951
  upper_lim_m4 = 210607
  upper_lim_m5 = 252595
  upper_lim_m6 = 96694
  vel_th_neg = -100
  vel_th_pos = 100
  x = 0
undefined symbols (not defined in the file): C, DiscIntNeverNeededParam
libraries: canmsglib x285, speedgoatlib_IO614 x245, simulink x26, slrealtimeloglib x9, simulink_extras x6, robotmaniplib x6
(part 1 of 13)
Description:
  | This model is to control the Hybrid_v2 via CAN protocol.
settings Model: SimulationMode=external  ExtModeEnableFloating=off  Creator=sbuccelli  LastModifiedBy=gbodo
settings SolverCC: ConcurrentTasks=on  AlgebraicLoopSolver=TrustRegion  PositivePriorityOrder=on  AutoInsertRateTranBlk=on
settings DataIOCC: SaveFormat=StructureWithTime
settings OptimizationCC: BlockReduction=off  OptimizeBlockIOStorage=off  BufferReuse=off  GlobalBufferReuse=off  ExpressionFolding=off  LocalBlockOutputs=off  OptimizeDataStoreBuffers=off  BusAssignmentInplaceUpdate=off
settings DebuggingCC: TasksWithSamePriorityMsg=none  UnconnectedInputMsg=warning  UnconnectedOutputMsg=warning  UnconnectedLineMsg=warning  SFMachineParentedDataDiag=warning
settings HardwareCC: ProdBitPerLong=64  ProdLongLongMode=on  ProdHWDeviceType=Intel->x86-64 (Linux 64)
settings ModelReferenceCC: EnableRefExpFcnMdlSchedulingChecks=on
settings RTWCC: Description=Simulink Real-Time  SystemTargetFile=slrealtime.tlc  TemplateMakefile=slrealtime_default_tmf  Toolchain=Simulink Real-Time Toolchain  BuildConfiguration=Faster Runs  CodeExecutionProfiling=on  TargetLang=C++  DLArmComputeVersion=19.05
settings CodeAppCC: MaxIdLength=95

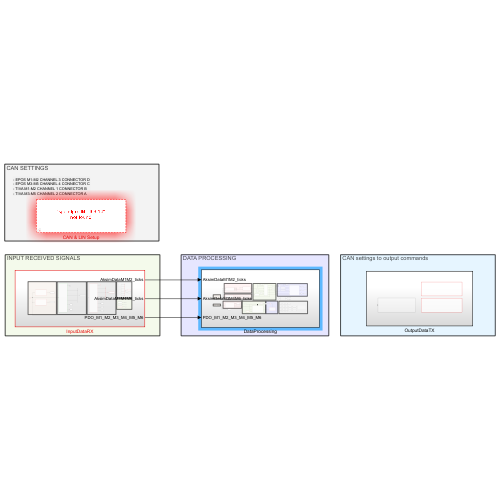
[thumbnail: Simulink's stored preview of the top-level diagram]
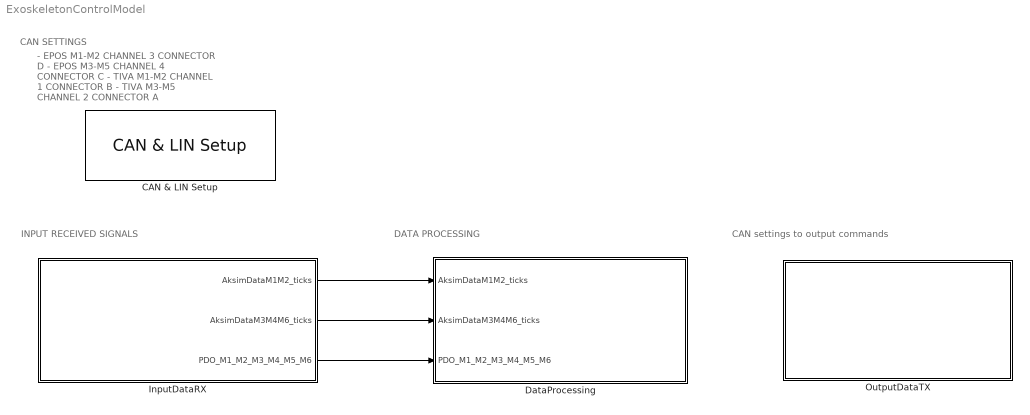
== system ExoskeletonControlModel ==
  note: INPUT RECEIVED SIGNALS
  note: - EPOS M1-M2 CHANNEL 3 CONNECTOR D
      | - EPOS M3-M5 CHANNEL 4 CONNECTOR C
      | - TIVA M1-M2 CHANNEL 1 CONNECTOR B
      | - TIVA M3-M5 CHANNEL 2 CONNECTOR A
  note: CAN SETTINGS
  note: DATA PROCESSING
  note: CAN settings to output commands
  CAN & LIN Setup : speedgoatlib_IO614/CAN & LIN Setup  id=1  drLtr=C:  PCISlot=-1  port1=CAN (HS/LS)  port2=CAN (HS)  port3=CAN (HS)  port4=CAN (HS)  opModeCAN1=Highspeed (HS)  bdrCAN1=1 MBaud  usrBdrCAN1=[5, 1, 13, 2]  stdAccMaskCAN1=[0, 0]  extAccMaskCAN1=[0, 0]  opModeCAN2=Highspeed (HS)  bdrCAN2=1 MBaud  usrBdrCAN2=[5, 1, 13, 2]  stdAccMaskCAN2=[0, 0]  extAccMaskCAN2=[0, 0]  opModeCAN3=Highspeed (HS)  bdrCAN3=1 MBaud  usrBdrCAN3=[5, 1, 13, 2]  stdAccMaskCAN3=[0, 0]  extAccMaskCAN3=[0, 0]  opModeCAN4=Highspeed (HS)  bdrCAN4=1 MBaud  usrBdrCAN4=[5, 1, 13, 2]  stdAccMaskCAN4=[0, 0]  extAccMaskCAN4=[0, 0]  initStruct=[]  termStruct=[]  opModeLIN=Master  bdrLIN=19200  protl=IO614  qtyMod=1  chNo=[1, 2, 3, 4]  ptTypes=[1, 1, 1, 1, 2]  protlHelpIdx=[0, 1, 2, 3, 0]  isFDMod=0  drvLtr=C:  opModeLIN2=Master  bdrLIN2=19200
  DataProcessing : Subsystem
  InputDataRX : Subsystem
  OutputDataTX : Subsystem
  wires:
  InputDataRX/1(AksimDataM1M2_ticks) -> DataProcessing/1(AksimDataM1M2_ticks)
  InputDataRX/2(AksimDataM3M4M6_ticks) -> DataProcessing/2(AksimDataM3M4M6_ticks)
  InputDataRX/3(PDO_M1_M2_M3_M4_M5_M6) -> DataProcessing/3(PDO_M1_M2_M3_M4_M5_M6)
